simulink model "Diff_Manchester"  (R2017b)
settings: Solver=ode45  StartTime=0.0  StopTime=2  RelTol=1e-3  AbsTol=1e-6
libraries: simulink_extras x2, commsequence2 x1
CloseFcn:
  | ;slview('closediagram',bdroot);
settings Model: ExtModeTrigMode=oneshot  ExtModeArmWhenConnect=off  Creator=cv  LastModifiedBy=cv
settings DataIOCC: SaveFormat=Array  SignalLoggingSaveFormat=ModelDataLogs  SignalLoggingName=sigsOut
settings OptimizationCC: BooleanDataType=off  InitFltsAndDblsToZero=on  LifeSpan=inf
settings DebuggingCC: SaveWithParameterizedLinksMsg=none  UnderspecifiedInitializationDetection=Classic  MergeDetectMultiDrivingBlocksExec=none  SignalResolutionControl=TryResolveAllWithWarning  MultiTaskDSMMsg=warning  MultiTaskCondExecSysMsg=none  FcnCallInpInsideContextMsg=warning  StrictBusMsg=None  SFUnexpectedBacktrackingDiag=warning  SFNoUnconditionalDefaultTransitionDiag=warning  SFExecutionAtInitializationDiag=none
settings HardwareCC: ProdBitPerPointer=32  ProdBitPerSizeT=32  ProdBitPerPtrDiffT=32  ProdLargestAtomicFloat=None  ProdIntDivRoundTo=Undefined  ProdEndianess=Unspecified  ProdWordSize=32  ProdHWDeviceType=32-bit Generic  TargetUnknown=on
settings ModelReferenceCC: PropagateSignalLabelsOutOfModel=off
settings RTWCC: Description=Generic Real-Time Target
settings CodeAppCC: StateflowObjectComments=on
settings GRTTargetCC: TargetFcnLib=ansi_tfl_tmw.mat  TargetLangStandard=C89/C90 (ANSI)  CombineOutputUpdateFcns=off  GRTInterface=on
settings ConfigComp: CovMetricSettings=dw  CovHtmlReporting=on  CovSaveCumulativeToWorkspaceVar=on  CovSaveSingleToWorkspaceVar=on  CovExternalEMLEnable=off

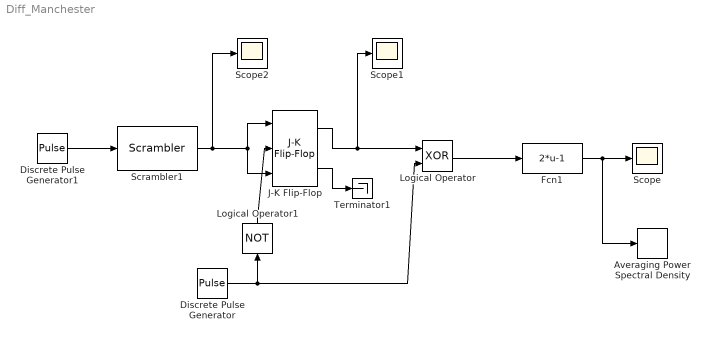
== system Diff_Manchester ==
  Averaging Power Spectral Density : simulink_extras/Additional Sinks/Averaging Power Spectral Density  npts=512  fftpts=4096  HowOften=256  sampleT=2*pi/80000
      link override sfunpsd: FunctionName=sfunpsd_mod  Parameters=fftpts,npts,HowOften,offset,ts,1,type_disp
      settings: SourceProductName=Simulink  SourceProductBaseCode=SL
  Discrete Pulse Generator : DiscretePulseGenerator  SampleTime=2*pi/20000
      settings: AttributesFormatString=CLK
  Discrete Pulse Generator1 : DiscretePulseGenerator  Period=8  SampleTime=2*pi/10000
      settings: AttributesFormatString=Data
  Fcn1 : Fcn  Expr=2*u-1
  J-K Flip-Flop : simulink_extras/Flip Flops/J-K Flip-Flop  initial_condition=0
      settings: SourceProductName=Simulink
  Logical Operator : Logic  Operator=XOR
  Logical Operator1 : Logic  Operator=NOT
  Scope : Scope
  Scope1 : Scope
  Scope2 : Scope
  Scrambler1 : commsequence2/Scrambler  M=2  poly=[0 -1 -7]  iniStaSource=Dialog Parameter  ini_sta=[1 1 1 1 1 1 1]  resetViaPort=off
      settings: SourceProductName=Communications System Toolbox  SourceProductBaseCode=CM
  Terminator1 : Terminator
  wires:
  Discrete Pulse Generator1/1 -> Scrambler1/1
  Scrambler1/1 -> Scope2/1, J-K Flip-Flop/1, J-K Flip-Flop/3
  Fcn1/1 -> Scope/1, Averaging Power Spectral Density/1
  Logical Operator/1 -> Fcn1/1
  J-K Flip-Flop/1 -> Scope1/1, Logical Operator/1
  Logical Operator1/1 -> J-K Flip-Flop/2
  J-K Flip-Flop/2 -> Terminator1/1
  Discrete Pulse Generator/1 -> Logical Operator1/1, Logical Operator/2
